simulink subsystem "jd2decYear"  (R2025b)
settings: Solver=VariableStepAuto  StartTime=0.0  StopTime=10.0  RelTol=1e-3
settings Model: Creator=antoniohernandez-rodiciomateos  LastModifiedBy=antoniohernandez-rodiciomateos

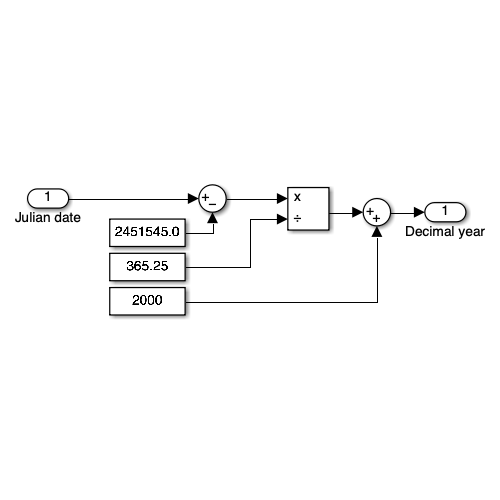
[thumbnail: Simulink's stored preview of the top-level diagram]
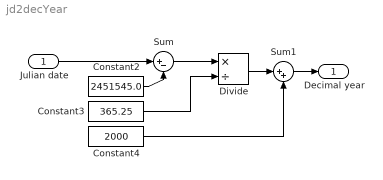
== system jd2decYear ==
  Julian date : Inport  OutDataTypeStr=double  PortDimensions=[1 1]
  Constant2 : Constant  Value=2451545.0
  Constant3 : Constant  Value=365.25
  Constant4 : Constant  Value=2000
  Divide : Product  Inputs=*/
  Sum : Sum  Inputs=|+-
  Sum1 : Sum  Inputs=|++
  Decimal year : Outport  OutDataTypeStr=double  PortDimensions=[1 1]
  wires:
  Constant3/1 -> Divide/2
  Constant2/1 -> Sum/2
  Sum/1 -> Divide/1
  Julian date/1 -> Sum/1
  Divide/1 -> Sum1/1
  Constant4/1 -> Sum1/2
  Sum1/1 -> Decimal year/1
